simulink model "ident_FOTD"  (R2024b)
settings: Solver=VariableStepAuto  StartTime=0.0  StopTime=10.0  RelTol=1e-3
values from neighbouring files (symbols this model uses):
  czas_skok = 20000    [ident.m]    (also in lab2.m = 10000)
  dPg = 0.1 * Pg0    (= 800)    [ident.m]    (also in lab2.m = 0)
  k = 4 / dPg    (= 0.005)    [ident.m]    (also in lab2.m = 1)
  T = 6.65 * 10000 - czas_skok    (= 46500)    [ident.m]    (also in lab2.m = 2190)
  T0 = 0.1 * T    (= 4650)    [ident.m]    (also in lab2.m = 37)
  Twew0 = (Pg0 + Tzew0*(cpp*rop*Fp0 + ((Ks*Kw)/(Kw + Ks)))) / (cpp*rop*Fp0 + ((Kw * Ks)/(Kw + Ks)))    (= 20)    [ident.m]    (also in lab2.m = 48.5714285714)
settings Model: Creator=Michal  LastModifiedBy=Michal
settings DataIOCC: ReturnWorkspaceOutputs=off

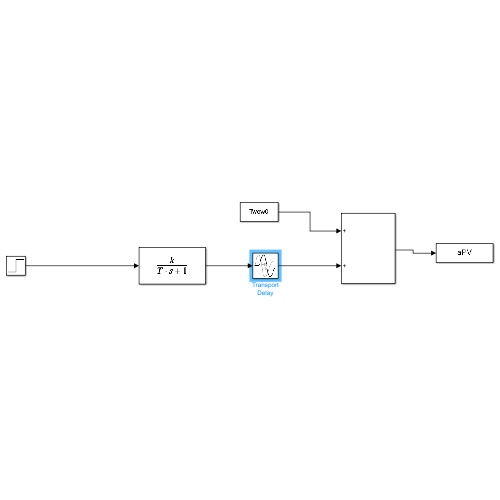
[thumbnail: Simulink's stored preview of the top-level diagram]
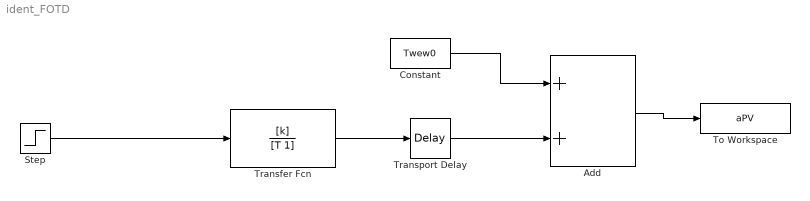
== system ident_FOTD ==
  Add : Sum
  Constant : Constant  Value=Twew0
  Step : Step  Time=czas_skok  After=dPg  SampleTime=0
  To Workspace : ToWorkspace  VariableName=aPV  SampleTime=-1
  Transfer Fcn : TransferFcn  Numerator=[k]  Denominator=[T 1]
  Transport Delay : TransportDelay  DelayTime=T0
  wires:
  Step/1 -> Transfer Fcn/1
  Transfer Fcn/1 -> Transport Delay/1
  Constant/1 -> Add/1
  Transport Delay/1 -> Add/2
  Add/1 -> To Workspace/1
